simulink model "goertzel_model"  (R2020b)
settings: Solver=VariableStepAuto  StartTime=0.0  StopTime=1  RelTol=1e-3
undefined symbols (not defined in the file or in its folder): j
settings Model: Creator=pablo  LastModifiedBy=pablo

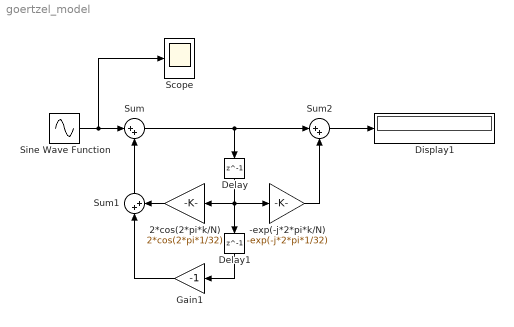
== system goertzel_model ==
  -exp(-j*2*pi*k/N) : Gain  Gain=-exp(-j*2*pi*1/32)
  2*cos(2*pi*k/N) : Gain  Gain=2*cos(2*pi*1/32)
  Delay : Delay  DelayLength=1  InitialCondition=0
  Delay1 : Delay  DelayLength=1  InitialCondition=0
  Display1 : Display
  Gain1 : Gain  Gain=-1
  Scope : Scope
  Sine Wave Function : Sin  SineType=Sample based  Samples=32  SampleTime=1/32
  Sum : Sum  Inputs=|++
  Sum1 : Sum  Inputs=|++
  Sum2 : Sum  Inputs=|++
  wires:
  Sum1/1 -> Sum/2
  2*cos(2*pi*k/N)/1 -> Sum1/2
  Delay/1 -> Delay1/1, 2*cos(2*pi*k/N)/1, -exp(-j*2*pi*k/N)/1
  Sum/1 -> Sum2/1, Delay/1
  Gain1/1 -> Sum1/1
  Delay1/1 -> Gain1/1
  -exp(-j*2*pi*k/N)/1 -> Sum2/2
  Sum2/1 -> Display1/1
  Sine Wave Function/1 -> Scope/1, Sum/1
